simulink model "LQG_ball"  (R2019b)
settings: Solver=VariableStepAuto  StartTime=0.0  StopTime=10.0  RelTol=1e-3
PostLoadFcn:
  | if any(exist('dsrtsu_mdlpostloadfcn', 'file') ~= 0), dsrtsu_mdlpostloadfcn('Execute', bdroot); end
InitFcn:
  | , if any(exist('rtifpga_mdlclblib', 'file') ~= 0), rtifpga_mdlclblib('Init', bdroot); end,
values from neighbouring files (symbols this model uses):
  ballLQRgain = lqr(ballSystem, Q, R)    [LQG_ball.m]    (also in LQG_plate_ball.m; LQR_ball.m)
  UseUserDefinedBallReference = 1    [LQG_ball.m]    (also in LQG_plate_ball.m; LQR_ball.m; PerformExperiment_CompareModelWithMeasurement.m = 0; Template_PerformExperiment.m = 0)
  UseUserDefinedPlateReference = 1    [LQG_ball.m]    (also in LQG_plate_ball.m; LQR_ball.m; PerformExperiment_CompareModelWithMeasurement.m; Template_PerformExperiment.m = 0)
  Ybop0 = [0.1;0;0;0]    [LQG_ball.m]    (also in LQG_plate_ball.m; LQR_ball.m)
undefined symbols (not defined in the file or in its folder): ballFFgain, Continuous, denc_mi, numc_mi, Time
libraries: ctrlSharedLib x1
settings Model: DSRTSU_INTERNAL_RTI_VER=570  DSRTSU_INTERNAL_RTI_TYPE=rti1202  RTICANMMDATA=struct('GeneralSetupData',struct('modelroot','C:\Users\20192433\Documents\SC-integration-project\Controllers','generalsettings',struct('filesettings',struct('destfolder',struct('Name','RTICANMM_FILES','Check',1),'buildfolder',struct('Name','.','Check',1),'AbsDestfolder',struct('Name','C:\Users\20192433\Documents\SC-integration-project\Controllers\RTICANMM_FILES'),'AbsBuildfolder',struct('Name','C:\Users\20192433\Documents\SC-integration-project\Controllers'))),'options',struct('addpaths',1,'rmpaths',1,'addtrcexclusion',true,'cannavigator',struct('checkmonitoring',0),'show_usrtrc',0,'use_usrtrc',0),'advanced',struct('options',ones(1,100)),'MPSetup',{{}},'RTI',struct('Type','RTI1202','Ver','7.15','Date','02-Nov-2020'),'modelname','LQG_ball','block','LQG_ball'))  DSRTSU_INTERNAL_RTIFPGA=170  Creator=Duin home  LastModifiedBy=Duin home

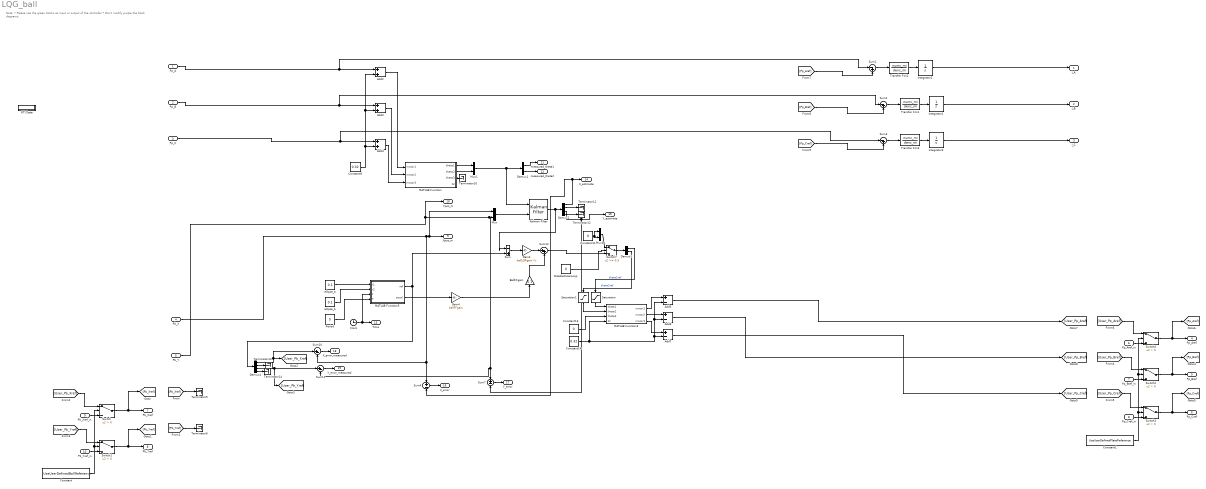
== system LQG_ball ==
  note: Note:
      | * Please use the green blocks as input or output of the controller
      | * Don't modify purple the block diagrams.
  Pp_A : Inport
  Pp_B : Inport  Port=2
  Pp_C : Inport  Port=3
  Pb_X : Inport  Port=4
  Pb_Y : Inport  Port=5
  Pp_Aref_in : Inport  Port=6
  Pp_Bref_in : Inport  Port=7
  Pp_Cref_in : Inport  Port=8
  Pb_Xref_in : Inport  Port=9
  Pb_Yref_in : Inport  Port=10
  Add2 : Sum
  Add3 : Sum
  Add4 : Sum
  Add5 : Sum  Inputs=+-
  Add6 : Sum  Inputs=+-
  Add7 : Sum  Inputs=+-
  BallFFgain : Gain  Gain=0.1
  Clock : Clock
  Constant : Constant  Value=UseUserDefinedBallReference
  Constant1 : Constant  Value=UseUserDefinedPlateReference
  Constant11 : Constant  Value=0
  Constant13 : Constant  Value=0
  Constant14 : Constant  Value=0.32
  Constant9 : Constant  Value=0.32
  Demux1 : Demux  Outputs=2
  Demux2 : Demux
  Demux3 : Demux  Outputs=2
  Demux4 : Demux
  "DisableOuterLoop " : Constant  Value=0
  Gain3 : Gain  Gain=ballLQRgain  Multiplication=Matrix(K*u)
  Gain4 : Gain  Gain=ballFFgain
  Integrator1 : Integrator  LimitOutput=on  UpperSaturationLimit=3  LowerSaturationLimit=-3
  Integrator2 : Integrator  LimitOutput=on  UpperSaturationLimit=3  LowerSaturationLimit=-3
  Integrator3 : Integrator  LimitOutput=on  UpperSaturationLimit=3  LowerSaturationLimit=-3
  Kalman Filter : ctrlSharedLib/Kalman Filter  TimeDomain=Continuous-Time  UseCurrentEstimator=on  ModelSource=LTI State-Space Variable  ModelSourceVariable=ballSystem  A=0.95  B=1  C=1  D=0  NumberOfStates=1  NumberOfInputs=1  NumberOfOutputs=1  InitialEstimateSource=Dialog  X0=Ybop0  P0=10  UseK=off  UseGH=off  NumberOfProcessNoiseInputs=1  G=1  TimeInvariantG=on  H=0  TimeInvariantH=on  Q=diag([1 20 1 20])  TimeInvariantQ=on  R=diag([0.02 0.02])  TimeInvariantR=on  N=0  TimeInvariantN=on  AddInputPort=on  AddEnablePort=off  OutputEstimatedY=off  OutputP=off  Ts=-1
      settings: SourceProductBaseCode=CT
  MATLAB Function : MATLAB Function  TreatAsAtomicUnit=on
  MATLAB Function3 : MATLAB Function  TreatAsAtomicUnit=on
  MATLAB Function5 : MATLAB Function  TreatAsAtomicUnit=on
  Mux : Mux  Inputs=2
  Mux1 : Mux  Inputs=2
  Mux4 : Mux  Inputs=2
  Period : Constant  Value=5
  RTI Data : Subsystem  Tag=struct('RTIDataServer',struct('RTIDataServerVs','2','RTIModelDescription','struct(''main'',''LQG_ball'',''sub'',''LQG_ball'',''isMp'',0)'))  LoadFcn="if exist('rtidc'), try,  rtidc('DataHostBlockClbLoad', gcbh); catch, disp(['Warning: ''LoadFcn'' for RTI Data block failed: ' lasterr]); end, end,"  mask(RTI_DATA_HOST){}
      mask help:
      | RTI Data Block.
      | This block is used by RTI to store internal model-dependent data.
      | Please keep this block on the root level of the model. Deleting this block will result in data loss.
      |
      | NEVER DELETE OR COPY THIS BLOCK!
      settings: CopyFcn="if exist('rtidc'), try,  rtidc('DataHostBlockClbCopy', gcbh); catch, disp(['Warning: ''CopyFcn'' for RTI Data block failed: ' lasterr]); end, end,"  DeleteFcn="if exist('rtidc'), try,  rtidc('DataHostBlockClbDelete', gcbh); catch, disp(['Warning: ''DeleteFcn'' for RTI Data block failed: ' lasterr]); end, end,"  ModelCloseFcn="if exist('rtidc'), try,  rtidc('DataHostBlockClbModelClose', gcbh); catch, disp(['Warning: ''ModelCloseFcn'' for RTI Data block failed: ' lasterr]); end, end,"  PreSaveFcn="if exist('rtidc'), try,  rtidc('DataHostBlockClbPreSave', gcbh); catch, disp(['Warning: ''PreSaveFcn'' for RTI Data block failed: ' lasterr]); end, end,"  PostSaveFcn="if exist('rtidc'), try,  rtidc('DataHostBlockClbPostSave', gcbh); catch, disp(['Warning: ''PostSaveFcn'' for RTI Data block failed: ' lasterr]); end, end,"  NameChangeFcn="if exist('rtidc'), try,  rtidc('DataHostBlockClbNameChange', gcbh); catch, disp(['Warning: ''NameChangeFcn'' for RTI Data block failed: ' lasterr]); end, end,"
      mask Help:
      | RTI Data Block.
      | This block is used by RTI to store internal model-dependent data.
      | Please keep this block on the root level of the model. Deleting this block will result in data loss.
      | 
      | NEVER DELETE OR COPY THIS BLOCK!
      mask Display:
      | text(0.5, 0.5, 'RTI Data', 'HorizontalAlignment', 'center');
      | plot([1 0]);
  Saturation : Saturate  UpperLimit=0.1  LowerLimit=-0.1
  Saturation1 : Saturate  UpperLimit=0.1  LowerLimit=-0.1
  Sum : Sum  Inputs=|-+
  Sum1 : Sum  Inputs=|-+  SaturateOnIntegerOverflow=on
  Sum10 : Sum  Inputs=|+-
  Sum11 : Sum  Inputs=|+-
  Sum12 : Sum  Inputs=|++
  Sum2 : Sum  Inputs=|-+  SaturateOnIntegerOverflow=on
  Sum3 : Sum  Inputs=|-+  SaturateOnIntegerOverflow=on
  Sum4 : Sum  Inputs=+-
  Sum7 : Sum  Inputs=+-
  Switch{,1..4} (5 alike) : Switch  Criteria=u2 > Threshold
  Switch7 : Switch  Threshold=0.5
  Terminator{5..6,10..14} (7 alike) : Terminator
  Transfer Fcn1 : TransferFcn  Numerator=numc_mi  Denominator=denc_mi
  Transfer Fcn2 : TransferFcn  Numerator=numc_mi  Denominator=denc_mi
  Transfer Fcn3 : TransferFcn  Numerator=numc_mi  Denominator=denc_mi
  ellipse_a : Constant  Value=0.1
  ellipse_b : Constant  Value=0.1
  I_A : Outport
  I_B : Outport  Port=2
  I_C : Outport  Port=3
  Pp_Aref : Outport  Port=4
  Pp_Bref : Outport  Port=5
  Pp_Cref : Outport  Port=6
  Pb_Xref : Outport  Port=7
  Pb_Yref : Outport  Port=8
  Xpos_m : Outport  Port=9
  Ypos_m : Outport  Port=10
  measured_theta1 : Outport  Port=11
  measured_theta2 : Outport  Port=12
  Time : Outport  Port=13
  X_estimate : Outport  Port=14
  Y_estimate : Outport  Port=15
  X_error : Outport  Port=16
  Y_error : Outport  Port=17
  X_error_measured : Outport  Port=18
  Y_error_measured : Outport  Port=19
  wires:
  Integrator1/1 -> I_B/1
  Integrator2/1 -> I_A/1
  Add7/1 -> [User_Pp_Cref]
  Add6/1 -> [User_Pp_Bref]
  Add5/1 -> [User_Pp_Aref]
  Pb_Xref_in/1 -> Switch/3
  Pb_Yref_in/1 -> Switch1/3
  Switch1/1 -> [Pb_Yref], Pb_Yref/1
  Switch/1 -> [Pb_Xref], Pb_Xref/1
  [User_Pb_Xref] -> Switch/1
  [User_Pb_Yref] -> Switch1/1
  Constant/1 -> Switch/2, Switch1/2
  Demux4/1 -> [User_Pb_Xref], Sum10/1
  Demux4/3 -> [User_Pb_Yref], Sum11/1
  [Pb_Yref] -> Terminator6/1
  [Pb_Xref] -> Terminator5/1
  Pp_Bref_in/1 -> Switch2/3
  [User_Pp_Bref] -> Switch2/1
  Switch3/1 -> [Pp_Cref], Pp_Cref/1
  Switch2/1 -> [Pp_Bref], Pp_Bref/1
  Pp_Cref_in/1 -> Switch3/3
  Constant1/1 -> Switch4/2, Switch2/2, Switch3/2
  [User_Pp_Cref] -> Switch3/1
  [User_Pp_Aref] -> Switch4/1
  Pp_Aref_in/1 -> Switch4/3
  Switch4/1 -> [Pp_Aref], Pp_Aref/1
  Mux1/1 -> Kalman Filter/1, Demux1/1
  MATLAB Function3/3(motor3) -> Add7/1
  MATLAB Function/2(theta2) -> Mux1/2
  Constant13/1 -> MATLAB Function3/3(theta3)
  Demux3/2 -> Saturation1/1  "theta2ref"
  MATLAB Function/3(theta3) -> Terminator10/1
  Add2/1 -> MATLAB Function/1(motor1)
  Add3/1 -> MATLAB Function/2(motor2)
  "DisableOuterLoop "/1 -> Switch7/2
  Constant11/1 -> Mux4/1, Mux4/2
  Sum11/1 -> Y_error_measured/1
  Clock/1 -> MATLAB Function5/3(t), Time/1
  Add4/1 -> MATLAB Function/3(motor3)
  Sum7/1 -> Y_error/1
  MATLAB Function/1(theta1) -> Mux1/1
  Mux/1 -> Kalman Filter/2
  Saturation/1 -> MATLAB Function3/1(theta1)
  BallFFgain/1 -> Sum12/2
  Saturation1/1 -> MATLAB Function3/2(theta2)
  Pb_Y/1 -> Ypos_m/1, Sum11/2, Sum7/1, Mux/2
  Demux2/4 -> Terminator12/1
  ellipse_b/1 -> MATLAB Function5/2(r2)
  Sum12/1 -> Switch7/3
  Sum/1 -> Gain3/1
  Demux2/1 -> X_estimate/1, Sum4/2
  Gain3/1 -> Sum12/1
  Demux4/4 -> Terminator14/1
  Demux3/1 -> Saturation/1  "theta1ref"
  Switch7/1 -> Demux3/1
  Sum10/1 -> X_error_measured/1
  MATLAB Function5/1(ref) -> Sum/2, Demux4/1
  MATLAB Function5/2(accel) -> Gain4/1
  Sum4/1 -> X_error/1
  Mux4/1 -> Switch7/1
  Demux4/2 -> Terminator13/1
  Demux2/3 -> Sum7/2, Y_estimate/1
  Demux2/2 -> Terminator11/1
  ellipse_a/1 -> MATLAB Function5/1(r1)
  MATLAB Function3/1(motor1) -> Add5/1
  Period/1 -> MATLAB Function5/4(T)
  Demux1/1 -> measured_theta1/1
  Gain4/1 -> BallFFgain/1
  Pb_X/1 -> Xpos_m/1, Mux/1, Sum10/2, Sum4/1
  Constant14/1 -> MATLAB Function3/4(Zc), Add7/2, Add6/2, Add5/2
  MATLAB Function3/2(motor2) -> Add6/1
  Kalman Filter/1 -> Sum/1, Demux2/1
  Demux1/2 -> measured_theta2/1
  Constant9/1 -> Add4/2, Add3/2, Add2/2
  [Pp_Aref] -> Sum1/2
  Pp_A/1 -> Sum1/1, Add2/1
  Transfer Fcn2/1 -> Integrator2/1
  Sum1/1 -> Transfer Fcn2/1
  Transfer Fcn1/1 -> Integrator1/1
  Pp_B/1 -> Sum2/1, Add3/1
  [Pp_Bref] -> Sum2/2
  Sum2/1 -> Transfer Fcn1/1
  Transfer Fcn3/1 -> Integrator3/1
  Pp_C/1 -> Sum3/1, Add4/1
  [Pp_Cref] -> Sum3/2
  Sum3/1 -> Transfer Fcn3/1
  Integrator3/1 -> I_C/1

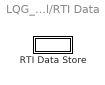
== system LQG_ball/RTI Data ==
  RTI Data Store : Subsystem  Tag=struct('private',struct('version',struct('dsVer',uint32(2),'dsVerCreation',uint32(2),'RTI',struct('ver','7.15','type','RTI1202')),'access',struct('type','Model','isPerm',1,'created',['25-Jun-2021 21:35:45'],'modified',['25-Jun-2021 22:49:53'],'location','')),'public',struct('main',struct('data',[]),'sub',struct('name','','data',[])))  mask(RTI_DATA_STORE){}
      mask help:
      | RTI Data Store Block. This block is used by RTI to store internal model dependent data. Deleting this block will result in data loss.
      |
      | NEVER DELETE, COPY, OR MODIFY THIS BLOCK!
      mask Help:
      | RTI Data Store Block. This block is used by RTI to store internal model dependent data. Deleting this block will result in data loss.
      | 
      | NEVER DELETE, COPY, OR MODIFY THIS BLOCK!
      mask Display: text(0.5, 0.5, ' ', 'HorizontalAlignment', 'center');

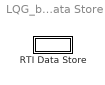
== system LQG_ball/RTI Data/RTI Data Store ==
  RTI Data Store : Subsystem  mask(RTI_DATA_STORE){}
      mask help:
      | RTI Data Store Block. This block is used by RTI to store internal model dependent data. Deleting this block will result in data loss.
      |
      | NEVER DELETE, COPY, OR MODIFY THIS BLOCK!
      mask Help:
      | RTI Data Store Block. This block is used by RTI to store internal model dependent data. Deleting this block will result in data loss.
      | 
      | NEVER DELETE, COPY, OR MODIFY THIS BLOCK!
      mask Display: text(0.5, 0.5, ' ', 'HorizontalAlignment', 'center');

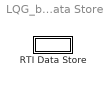
== system LQG_ball/RTI Data/RTI Data Store/RTI Data Store ==
  RTI Data Store : Subsystem  mask(RTI_DATA_STORE){}
      mask help:
      | RTI Data Store Block. This block is used by RTI to store internal model dependent data. Deleting this block will result in data loss.
      |
      | NEVER DELETE, COPY, OR MODIFY THIS BLOCK!
      mask Help:
      | RTI Data Store Block. This block is used by RTI to store internal model dependent data. Deleting this block will result in data loss.
      | 
      | NEVER DELETE, COPY, OR MODIFY THIS BLOCK!
      mask Display: text(0.5, 0.5, ' ', 'HorizontalAlignment', 'center');

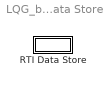
== system LQG_ball/RTI Data/RTI Data Store/RTI Data Store/RTI Data Store ==
  RTI Data Store : Subsystem  mask(RTI_DATA_STORE){}
      mask help:
      | RTI Data Store Block. This block is used by RTI to store internal model dependent data. Deleting this block will result in data loss.
      |
      | NEVER DELETE, COPY, OR MODIFY THIS BLOCK!
      mask Help:
      | RTI Data Store Block. This block is used by RTI to store internal model dependent data. Deleting this block will result in data loss.
      | 
      | NEVER DELETE, COPY, OR MODIFY THIS BLOCK!
      mask Display: text(0.5, 0.5, ' ', 'HorizontalAlignment', 'center');

== system LQG_ball/RTI Data/RTI Data Store/RTI Data Store/RTI Data Store/RTI Data Store ==

== matlab function LQG_ball/MATLAB Function ==
  data: motor1 input; theta1 output; motor2 input; motor3 input; theta2 output; theta3 output; Zc output
% Roll-Pitch-Yaw angles to motors position
% Roll (theta1): rotation about x-axis
% Pitch (theta2): rotation about y-axis
% Yaw (theta3): rotation about z-axis
% See page 12 and Appendix A (Multibody and Nonlinear Dynamics lecture
% notes for further reference
% Motors (1,2,3) -> (A,B,C)

function [theta1,theta2,theta3,Zc] = motorsToAngles2(motor1, motor2, motor3)

%% Define parameters
r = 0.17;
r0B1 = [r; 0; 0];      
r0B2 = [-0.5*r; (sqrt(3)/2)*r; 0];
r0B3 = [-0.5*r; -(sqrt(3)/2)*r; 0];
r0B = [r0B1 r0B2 r0B3];
%r1C1 = r0B1; r1C2 = r0B2; r1C3 = r0B3;
r1C = r0B;

%% Find Zc
Zc = 1/3*(motor1+motor2+motor3);
r0Oc = [0;0;Zc];

%% Assemble matrices
rBC = [0 0 0; 0 0 0; motor1 motor2 motor3];
r0OC = [r0Oc r0Oc r0Oc];

%% Find A10 (Using \ operator to solve a system of linear equation since the matrix r1C is singular)
CPi_rotated = rBC+r0B-r0OC;
P1b = CPi_rotated(:,1);
P2b = CPi_rotated(:,2);
P3b = CPi_rotated(:,3);

%base frame unit vectors
UnitX=[1;0;0];
UnitY=[0;1;0];
UnitZ=[0;0;1];
UnitXp=P1b/sqrt(dot(P1b,P1b));
UnitZp=cross(UnitXp,P3b);
UnitZp=UnitZp/sqrt(dot(UnitZp,UnitZp)); %now length 1
UnitYp=cross(UnitXp,UnitZp);

theta2=asin(-UnitXp(3));
theta3=asin(UnitXp(2)/sqrt(1-UnitXp(3)^2));
theta1=asin(UnitYp(3)/sqrt(1-UnitXp(3)^2));

end

== matlab function LQG_ball/MATLAB Function3 ==
  data: theta1 input; motor1 output; theta2 input; theta3 input; Zc input; motor2 output; motor3 output
% Roll-Pitch-Yaw angles to motors position
% Roll (theta1): rotation about x-axis
% Pitch (theta2): rotation about y-axis
% Yaw (theta3): rotation about z-axis
% See page 12 and Appendix A (Multibody and Nonlinear Dynamics lecture
% notes for further reference
% Motors (1,2,3) -> (A,B,C)

function [motor1, motor2, motor3] = anglesToMotors(theta1,theta2,theta3,Zc)

%% Define parameters
r = 0.17;
r0B1 = [r; 0; 0];      
r0B2 = [-0.5*r; (sqrt(3)/2)*r; 0];
r0B3 = [-0.5*r; -(sqrt(3)/2)*r; 0];
r0B = [r0B1 r0B2 r0B3];
%r1C1 = r0B1; r1C2 = r0B2; r1C3 = r0B3;
r1C = r0B;
r0Oc = [0;0;Zc];

% Find cos and sin to accelerate calculations
C1 = cos(theta1);S1 = sin(theta1);C2 = cos(theta2);S2 = sin(theta2);C3 = cos(theta3);S3 = sin(theta3);

% Rotation matrices
RotZ = [C3 S3 0; -S3 C3 0; 0 0 1];
RotY = [C2 0 -S2; 0 1 0; S2 0 C2];
RotX = [1 0 0; 0 C1 S1; 0 -S1 C1];

A10 = RotX*RotY*RotZ; A01 = A10';

% Find rCiBi (Vectors representing the motors)
rCiBi = zeros(3,3);
for i=1:3
    rCiBi(:,i) = r0Oc + A01*r1C(:,i) - r0B(:,i);
end

% Outputs to motor are the lengths of the vectors
motor1 = norm(rCiBi(:,1));
motor2 = norm(rCiBi(:,2));
motor3 = norm(rCiBi(:,3));
end

== matlab function LQG_ball/MATLAB Function5 ==
  data: r1 input; ref output; r2 input; t input; T input; accel output
function [ref,accel] = refGenerator(r1,r2,t,T)
omega = 2*pi/T;
x = r1*sin(omega*t);
xdot = r1*omega*cos(omega*t);
xddot = -r1*omega^2*sin(omega*t);
y = r2*cos(omega*t);
ydot = -r2*omega*sin(omega*t);
yddot = -r2*omega^2*cos(omega*t);
ref = [x;xdot;y;ydot];
accel = [yddot;xddot];
end
